simulink model "mcp4822_task"  (Simulink 3.00)
libraries: mathlib x4, speclib x1

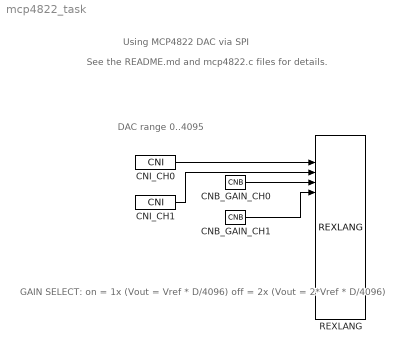
== system mcp4822_task ==
  note: DAC range 0..4095
  note: Using MCP4822 DAC via SPI
  note: See the README.md and mcp4822.c files for details.
  note: GAIN SELECT:
      | on = 1x (Vout = Vref * D/4096)
      | off = 2x (Vout = 2*Vref * D/4096)
  CNB_GAIN_CH0 : mathlib/CNB  YCN=on
  CNB_GAIN_CH1 : mathlib/CNB  YCN=on
  CNI_CH0 : mathlib/CNI  icn=2047
  CNI_CH1 : mathlib/CNI  icn=500
  REXLANG : speclib/REXLANG  strs=0  srcname=mcp4822.c  srctype=1: C-like  stack=0  debug=1: No check  fname=/dev/spidev0.0  p0=/dev/spidev0.0
  wires:
  CNB_GAIN_CH0/1 -> REXLANG/5
  CNB_GAIN_CH1/1 -> REXLANG/6
  CNI_CH0/1 -> REXLANG/3
  CNI_CH1/1 -> REXLANG/4
